simulink library "IR_varmeeffekt_function"  (R2025b)
settings: Solver=VariableStepAuto  StartTime=0.0  StopTime=10.0  RelTol=1e-3
settings Model: Creator=cdt  LastModifiedBy=cdt

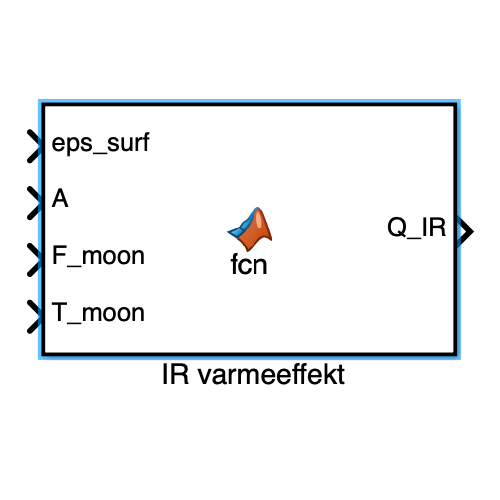
[thumbnail: Simulink's stored preview of the top-level diagram]
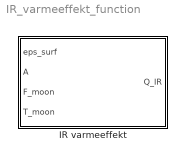
== system IR_varmeeffekt_function ==
  " IR varmeeffekt" : MATLAB Function  TreatAsAtomicUnit=on

== matlab function IR_varmeeffekt_function/ IR varmeeffekt ==
  data: Q_IR output; eps_surf input; A input; F_moon input; T_moon input
function Q_IR = fcn(eps_surf, A, F_moon, T_moon)
% Q_IR: total absorberet infrarød varmeeffekt fra månen (W)
% eps_surf: IR-emissivitet (absorptans) af roverens overflade
% A: areal af roverens overflade (m^2)
% F_moon: view factor til månen (0 til 1)
% T_moon: månens lokale overfladetemperatur (K)


sigma = 5.670e-8; % Stefan-Boltzmann konstant (W/(m^2*K^4))
eps_moon = 0.95; % månens emissivitet

% Beregn den absorberede infrarøde varmestråling fra måneoverfladen
Q_IR = eps_surf * sigma * A * eps_moon * F_moon * (T_moon)^4;
